simulink model "EEL_5661_F21_bicycle_092121"  (R2019a)
settings: Solver=VariableStepAuto  StartTime=0.0  StopTime=10.0  RelTol=1e-3
libraries: simulink x1
settings Model: Creator=rothz  LastModifiedBy=rothz

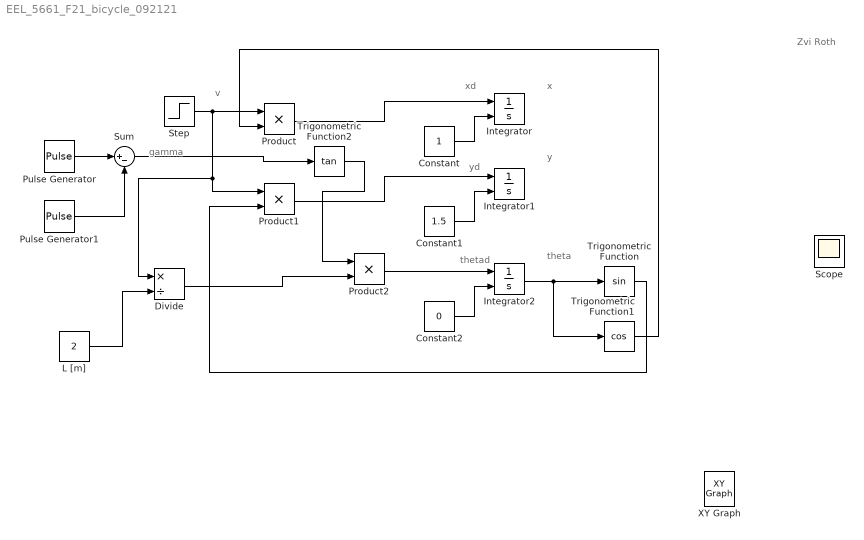
== system EEL_5661_F21_bicycle_092121 ==
  note: gamma
  note: v
  note: thetad
  note: yd
  note: xd
  note: theta
  note: y
  note: x
  note: Zvi Roth
  Constant : Constant
  Constant1 : Constant  Value=1.5
  Constant2 : Constant  Value=0
  Divide : Product  Inputs=*/
  Integrator : Integrator  InitialConditionSource=external
  Integrator1 : Integrator  InitialConditionSource=external
  Integrator2 : Integrator  InitialConditionSource=external
  L [m] : Constant  Value=2
  Product : Product
  Product1 : Product
  Product2 : Product
  Pulse Generator : DiscretePulseGenerator  PulseType=Time based  Period=10  PulseWidth=5
  Pulse Generator1 : DiscretePulseGenerator  PulseType=Time based  Period=10  PulseWidth=5
  Scope : Scope
  Step : Step  SampleTime=0
  Sum : Sum  Inputs=|+-
  Trigonometric Function : Trigonometry
  Trigonometric Function1 : Trigonometry  Operator=cos
  Trigonometric Function2 : Trigonometry  Operator=tan
  XY Graph : simulink/Sinks/XY Graph  xmin=-1  xmax=1  ymin=-1  ymax=1  st=-1
  wires:
  Constant/1 -> Integrator/2
  Constant1/1 -> Integrator1/2
  Constant2/1 -> Integrator2/2
  Integrator2/1 -> Trigonometric Function1/1, Trigonometric Function/1
  Step/1 -> Divide/1, Product1/1, Product/1
  Trigonometric Function1/1 -> Product/2
  Product/1 -> Integrator/1
  Trigonometric Function/1 -> Product1/2
  Product1/1 -> Integrator1/1
  Pulse Generator/1 -> Sum/1
  Pulse Generator1/1 -> Sum/2
  L [m]/1 -> Divide/2
  Sum/1 -> Trigonometric Function2/1
  Divide/1 -> Product2/2
  Trigonometric Function2/1 -> Product2/1
  Product2/1 -> Integrator2/1
